simulink library "Lib_DQTrans_dqs2abc"  (R2021a)
settings: Solver=VariableStepAuto  StartTime=0.0  StopTime=10.0  RelTol=1e-3
undefined symbols (not defined in the file): C_SQRT3
settings Model: Creator=30610  LastModifiedBy=30610

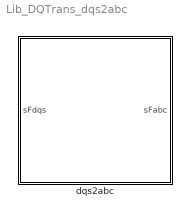
== system Lib_DQTrans_dqs2abc ==
  dqs2abc : Subsystem

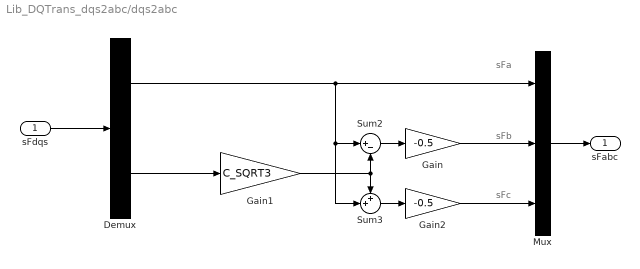
== system Lib_DQTrans_dqs2abc/dqs2abc ==
  note: sFc
  note: sFb
  note: sFa
  sFdqs : Inport
  Demux : Demux  Outputs=2
  Gain : Gain  Gain=-0.5
  Gain1 : Gain  Gain=C_SQRT3
  Gain2 : Gain  Gain=-0.5
  Mux : Mux  Inputs=3
  Sum2 : Sum  Inputs=|+-
  Sum3 : Sum  Inputs=++|
  sFabc : Outport  VectorParamsAs1DForOutWhenUnconnected=off
  wires:
  Gain2/1 -> Mux/3
  Sum3/1 -> Gain2/1
  Demux/1 -> Mux/1, Sum3/2, Sum2/1
  Sum2/1 -> Gain/1
  Mux/1 -> sFabc/1
  Gain/1 -> Mux/2
  Demux/2 -> Gain1/1
  Gain1/1 -> Sum3/1, Sum2/2
  sFdqs/1 -> Demux/1
